simulink model "electrolyser_v3"  (R2021b)
settings: Solver=VariableStepAuto  StartTime=0.0  StopTime=10.0  RelTol=1e-3
model workspace: external: MATLAB File parameters_SS.m (data not in the file)
values from neighbouring files (symbols this model uses):
  clnt =     [output_serpentine.mat]    (also in output_straight.mat)
  const =     [const.mat]    (also in output_serpentine.mat; output_straight.mat)
  pemel =     [output_serpentine.mat]    (also in output_straight.mat)
libraries: fl_lib x29, nesl_utility x7, SimscapeFluids_lib x3
(part 2 of 2)

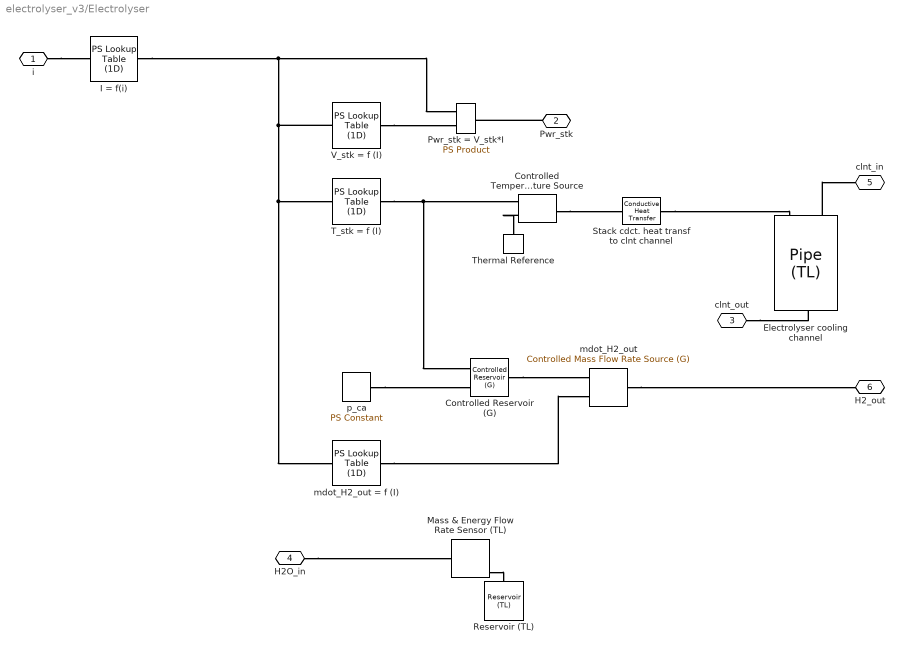
== system electrolyser_v3/Electrolyser ==
  Controlled Temperature Source : fl_lib/Thermal/Thermal Sources/Controlled Temperature Source
  Controlled Reservoir (G) : fl_lib/Gas/Elements/Controlled Reservoir (G)  area_A=pemel.totAc_ch_stk m^2
      settings: SourceProductBaseCode=SS  InternalSimscapePortConfiguration="{\"Bottom\":[],\"Left\":[{\"id\":\"A\",\"label\":\"A\",\"type\":\"foundation.gas.gas\"}],\"Right\":[{\"id\":\"T_in\",\"label\":\"T\",\"type\":\"input\"},{\"id\":\"p_in\",\"label\":\"P\",\"type\":\"input\"}],\"Top\":[]}"
  Electrolyser cooling channel : SimscapeFluids_lib/Thermal Liquid/Pipes & Fittings/Pipe (TL)  dynamic_compressibility=simscape.enum.onoff.off  inertia=simscape.enum.onoff.off  num_segments=1  pipe_length=pemel.L_clt m  area=pemel.totAc_clt_stk m^2  Dh=pemel.Dh_clt m  wall_spec=fluids.thermal_liquid.pipes_fittings.enum.wall_spec.rigid  Dh_rigid=0.1128 m  wall_compliance=1.2e-6 m/MPa  wall_time_constant=0.01 s  elevation_spec=foundation.enum.constant_variable.constant  elevation_gain=0 m  g=9.81 m/s^2  pressure_loss_spec=fluids.thermal_liquid.pipes_fittings.enum.PressureLossSpec.Nominal  length_add=1 m  roughness=15e-6 m  Re_friction_TLU=[400, 1000, 1500, 3000, 4000, 6000, 10000, 20000, 40000, 60000, 100000, 100000000]  friction_factor_TLU=[.264, .112, .071, .0417, .0387, .0268, .025, .0232, .0226, .022, .0214, .0214]  shape_factor=64  Re_lam=2000  Re_tur=4000  mdot_nominal=clnt.mdot_stk kg/s  p_diff_nominal=clnt.dp_stk Pa  mdot_threshold=1e-12 kg/s  heat_transfer_spec=fluids.thermal_liquid.pipes_fittings.enum.HeatTransferSpec.Nominal  mdot_nominal_heat=clnt.mdot_stk kg/s  T_in_nominal=clnt.T_stk_in K  T_out_nominal=clnt.T_stk_in + clnt.dT_stk K  p_in_nominal_heat=clnt.p_stk_in Pa  T_wall_nominal=pemel.T_stk K  a_coeff=0.023  b_Re_power=0.8  c_Pr_power=0.4  Nu_lam=3.66  Re_Colburn_TLU=[100, 150, 1000]  Colburn_factor_TLU=[.019, .013, .002]  Re_Nu_TLU=[100, 150, 1000]  Pr_Nu_TLU=[1, 10]  Nu_TLU=[3.72, 4.21; 3.75, 4.44; 4.21, 7.15]  T0_vec=amb.T K  p0_vec=0.101325 MPa  mdot0=0.1 kg/s
      settings: SourceProductBaseCode=SH
  I = f(i) : fl_lib/Physical Signals/Lookup Tables/PS Lookup Table (1D)  x=pemel.i_i A/cm^2  f=pemel.I_i A  interp_method=simscape.enum.interpolation.linear  extrap_method=simscape.enum.extrapolation.linear
      settings: SourceProductBaseCode=SS
  Mass & Energy Flow Rate Sensor (TL) : fl_lib/Thermal Liquid/Sensors/Mass & Energy Flow Rate Sensor (TL)
      settings: SourceProductBaseCode=SS  InternalSimscapePortConfiguration="{\"Bottom\":[],\"Left\":[{\"id\":\"A\",\"label\":\"A\",\"type\":\"foundation.thermal_liquid.thermal_liquid\"}],\"Right\":[{\"id\":\"B\",\"label\":\"B\",\"type\":\"foundation.thermal_liquid.thermal_liquid\"},{\"id\":\"M\",\"label\":\"M\",\"type\":\"output\"},{\"id\":\"PHI\",\"label\":\"Phi\",\"type\":\"output\"}],\"Top\":[]}"
  Pwr_stk = V_stk*I : fl_lib/Physical Signals/Functions/PS Product
  Reservoir (TL) : fl_lib/Thermal Liquid/Elements/Reservoir (TL)  pressure_spec=foundation.enum.pressure_spec.atmospheric  reservoir_pressure=0.101325 MPa  reservoir_temperature=293.15 K  area=0.01 m^2
      settings: SourceProductBaseCode=SS
  Stack cdct. heat transf to clnt channel : fl_lib/Thermal/Thermal Elements/Conductive Heat Transfer  area=pemel.Prm_clt*pemel.L_clt m^2  thickness=0.001 m  th_cond=50 W/(m*K)  T_specify=off  T_priority=None  T=0 K  T_nominal_specify=off  T_nominal_unit=K  T_nominal_value=1  Q_specify=off  Q_priority=None  Q=0 W  Q_nominal_specify=off  Q_nominal_unit=W  Q_nominal_value=1
  T_stk = f (I) : fl_lib/Physical Signals/Lookup Tables/PS Lookup Table (1D)  x=pemel.I_i A  f=pemel.T_i K  interp_method=simscape.enum.interpolation.smooth  extrap_method=simscape.enum.extrapolation.linear
      settings: SourceProductBaseCode=SS
  Thermal Reference : fl_lib/Thermal/Thermal Elements/Thermal Reference
  V_stk = f (I) : fl_lib/Physical Signals/Lookup Tables/PS Lookup Table (1D)  x=pemel.I_i A  f=pemel.V_stk_i V  interp_method=simscape.enum.interpolation.smooth  extrap_method=simscape.enum.extrapolation.linear
      settings: SourceProductBaseCode=SS
  mdot_H2_out : fl_lib/Gas/Sources/Controlled Mass Flow Rate Source (G)  power_spec=foundation.enum.power_spec.isentropic  area_A=pemel.Ac_ch m^2  area_B=pemel.Ac_ch m^2
      settings: SourceProductBaseCode=SS  InternalSimscapePortConfiguration="{\"Bottom\":[],\"Left\":[{\"id\":\"A\",\"label\":\"A\",\"type\":\"foundation.gas.gas\"},{\"id\":\"M\",\"label\":\"M\",\"type\":\"input\"}],\"Right\":[{\"id\":\"B\",\"label\":\"B\",\"type\":\"foundation.gas.gas\"}],\"Top\":[]}"
  mdot_H2_out = f (I) : fl_lib/Physical Signals/Lookup Tables/PS Lookup Table (1D)  x=pemel.I_i A  f=pemel.H2out_i kg/s  interp_method=simscape.enum.interpolation.smooth  extrap_method=simscape.enum.extrapolation.linear
      settings: SourceProductBaseCode=SS
  p_ca : fl_lib/Physical Signals/Sources/PS Constant  constant=pemel.p_ca
  i : PMIOPort  Side=Left
  Pwr_stk : PMIOPort  Port=2  Side=Right
  clnt_out : PMIOPort  Port=3  Side=Left
  H2O_in : PMIOPort  Port=4  Side=Left
  clnt_in : PMIOPort  Port=5  Side=Right
  H2_out : PMIOPort  Port=6  Side=Right
  connections:
  mdot_H2_out/RConn1 -- H2_out/RConn1
  H2O_in/RConn1 -- Mass & Energy Flow Rate Sensor (TL)/LConn1
  clnt_out/RConn1 -- Electrolyser cooling channel/RConn1
  Electrolyser cooling channel/LConn1 -- clnt_in/RConn1
  V_stk = f (I)/RConn1 -- Pwr_stk = V_stk*I/LConn2
  Pwr_stk/RConn1 -- Pwr_stk = V_stk*I/RConn1
  Controlled Temperature Source/LConn1 -- Stack cdct. heat transf to clnt channel/LConn1
  Stack cdct. heat transf to clnt channel/RConn1 -- Electrolyser cooling channel/LConn2
  T_stk = f (I)/RConn1 -- Controlled Reservoir (G)/RConn1 -- Controlled Temperature Source/RConn1
  Controlled Temperature Source/RConn2 -- Thermal Reference/LConn1
  Controlled Reservoir (G)/LConn1 -- mdot_H2_out/LConn1
  p_ca/RConn1 -- Controlled Reservoir (G)/RConn2
  mdot_H2_out = f (I)/RConn1 -- mdot_H2_out/LConn2
  I = f(i)/RConn1 -- T_stk = f (I)/LConn1 -- mdot_H2_out = f (I)/LConn1 -- V_stk = f (I)/LConn1 -- Pwr_stk = V_stk*I/LConn1
  i/RConn1 -- I = f(i)/LConn1
  Mass & Energy Flow Rate Sensor (TL)/RConn1 -- Reservoir (TL)/LConn1
